simulink model "labTHREEtaskTWO"  (R2023b)
settings: Solver=VariableStepAuto  StartTime=0.0  StopTime=10  RelTol=1e-3
libraries: simulink x2, dspfdesign x1, commsynccomp2 x1
settings Model: Creator=omarf  LastModifiedBy=omarf

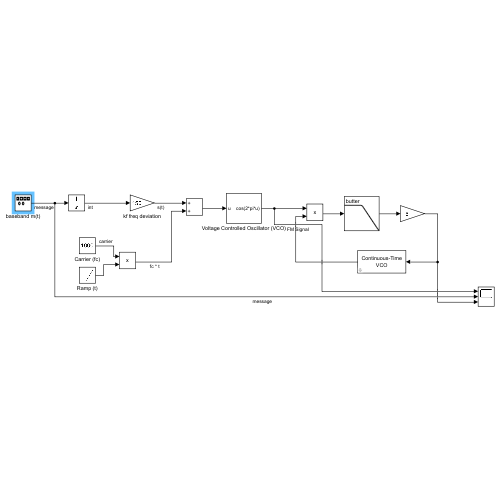
[thumbnail: Simulink's stored preview of the top-level diagram]
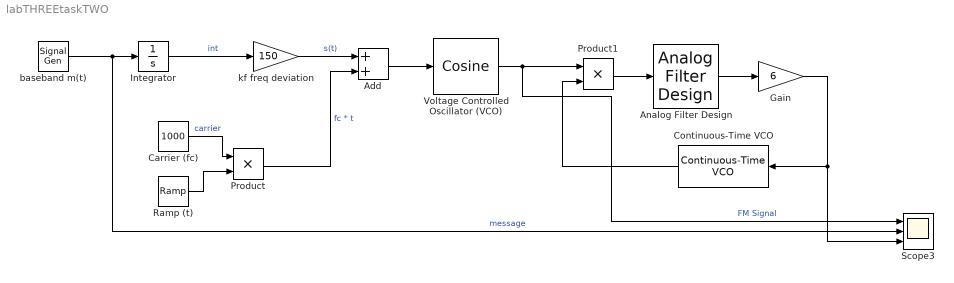
== system labTHREEtaskTWO ==
  Add : Sum
  Analog Filter Design : dspfdesign/Analog Filter Design  method=Butterworth  filttype=Lowpass  N=8  Wlo=630  Whi=80  Rp=2  Rs=40
  Carrier (fc) : Constant  Value=1000
  Continuous-Time VCO : commsynccomp2/Continuous-Time VCO  Ac=1  Fc=1000  Kc=1  Ph=0
  Gain : Gain  Gain=6
  Integrator : Integrator
  Product : Product
  Product1 : Product
  Ramp (t) : simulink/Sources/Ramp  slope=1  start=0  InitialOutput=0
  Scope3 : Scope  NumInputPorts=3
  Voltage Controlled Oscillator (VCO) : simulink/Lookup Tables/Cosine  Formula=cos(2*pi*u)  NumDataPoints=(2^5)+1  OutputWordLength=16  InternalRulePriority=Speed
  baseband m(t) : SignalGenerator  Amplitude=2  Frequency=100*2*pi  Units=rad/sec
  kf freq deviation : Gain  Gain=150
  wires:
  Carrier (fc)/1 -> Product/1  "carrier"
  baseband m(t)/1 -> Scope3/2, Integrator/1  "message"
  Integrator/1 -> kf freq deviation/1  "int"
  kf freq deviation/1 -> Add/1  "s(t)"
  Ramp (t)/1 -> Product/2
  Product/1 -> Add/2  "fc * t"
  Add/1 -> Voltage Controlled Oscillator (VCO)/1
  Voltage Controlled Oscillator (VCO)/1 -> Scope3/1, Product1/1  "FM Signal"
  Product1/1 -> Analog Filter Design/1
  Analog Filter Design/1 -> Gain/1
  Gain/1 -> Continuous-Time VCO/1, Scope3/3
  Continuous-Time VCO/1 -> Product1/2
